simulink model "robotGrasper_FSFwInt"  (R2020a)
settings: Solver=ode45  StartTime=0.0  StopTime=tend  FixedStep=.000001  RelTol=1e-3
values from neighbouring files (symbols this model uses):
  c1 = 9982    [Robot_Grasper.m]
  c2 = -2871    [Robot_Grasper.m]
  d = 3.1    [Robot_Grasper.m]
  i_MAX = 10    [Robot_Grasper.m]
  K_FSFwInt = [Ki(1) Ki(2)]    [Robot_Grasper.m]
  Ke = -Ki(3)    [Robot_Grasper.m]
  KtKm = 1e-3*11.3    (= 0.0113)    [Robot_Grasper.m]
  m = 0.5    [Pendulum_Controller.m]    (also in Robot_Grasper.m = 0.155)
undefined symbols (not defined in the file or in its folder): a, c3
settings Model: Creator=pjseiler  LastModifiedBy=ye000064
settings DataIOCC: LimitDataPoints=on  SaveFormat=Array  ReturnWorkspaceOutputs=off
settings OptimizationCC: BlockReduction=off  BooleanDataType=off  LifeSpan=inf
settings DebuggingCC: SaveWithParameterizedLinksMsg=none  UnderspecifiedInitializationDetection=Classic  MergeDetectMultiDrivingBlocksExec=none  SignalResolutionControl=TryResolveAllWithWarning  SFUnexpectedBacktrackingDiag=warning  SFNoUnconditionalDefaultTransitionDiag=warning  SFExecutionAtInitializationDiag=none  ArithmeticOperatorsInVariantConditions=warning
settings HardwareCC: ProdBitPerPointer=32  ProdBitPerSizeT=32  ProdBitPerPtrDiffT=32  ProdLargestAtomicFloat=None  ProdIntDivRoundTo=Undefined  ProdEndianess=Unspecified  ProdWordSize=32  ProdHWDeviceType=32-bit Generic  TargetUnknown=on
settings ModelReferenceCC: PropagateSignalLabelsOutOfModel=off
settings SFSimCC: SimUseLocalCustomCode=off  CustomCodeUndefinedFunction=UseInterfaceOnly
settings RTWCC: RTWUseLocalCustomCode=off
settings CodeAppCC: StateflowObjectComments=on
settings GRTTargetCC: TargetLangStandard=C89/C90 (ANSI)
settings ConfigComp: CovMetricSettings=dw  CovHtmlReporting=on  CovSaveCumulativeToWorkspaceVar=on  CovSaveSingleToWorkspaceVar=on  CovExternalEMLEnable=off  CovSFcnEnable=off

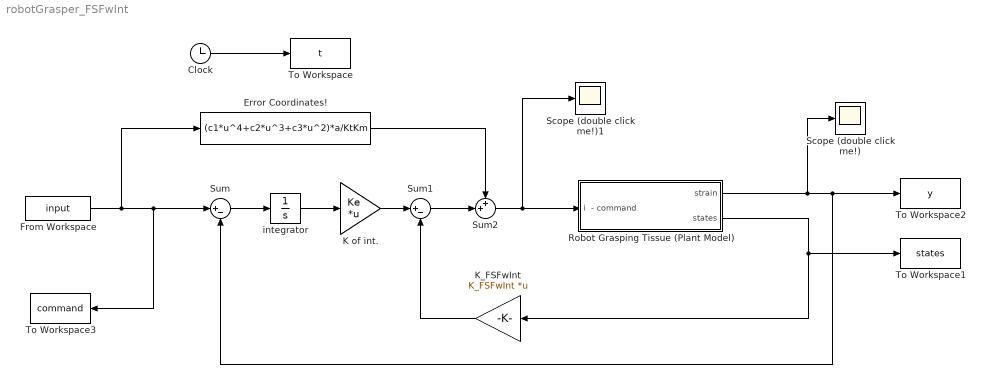
== system robotGrasper_FSFwInt ==
  Clock : Clock
  Error Coordinates! : Fcn  Expr=(c1*u^4+c2*u^3+c3*u^2)*a/KtKm
  From Workspace : FromWorkspace  VariableName=input
  K of int. : Gain  Gain=Ke  Multiplication=Matrix(K*u)
  K_FSFwInt : Gain  Gain=K_FSFwInt  Multiplication=Matrix(K*u)
  "Robot Grasping Tissue (Plant Model) " : Subsystem
  Scope (double click me!) : Scope
  Scope (double click me!)1 : Scope
  Sum : Sum  Inputs=|+-
  Sum1 : Sum  Inputs=|+-
  Sum2 : Sum  Inputs=++|
  To Workspace : ToWorkspace  VariableName=t  SampleTime=-1
  To Workspace1 : ToWorkspace  VariableName=states  SampleTime=-1
  To Workspace2 : ToWorkspace  VariableName=y  SampleTime=-1
  To Workspace3 : ToWorkspace  VariableName=command  SampleTime=-1
  integrator : Integrator
  wires:
  "Robot Grasping Tissue (Plant Model) "/1("strain ") -> To Workspace2/1, Sum/2, Scope (double click me!)/1
  Clock/1 -> To Workspace/1
  integrator/1 -> K of int./1
  Sum/1 -> integrator/1
  K of int./1 -> Sum1/1
  K_FSFwInt/1 -> Sum1/2
  "Robot Grasping Tissue (Plant Model) "/2(states) -> K_FSFwInt/1, To Workspace1/1
  From Workspace/1 -> Error Coordinates!/1, Sum/1, To Workspace3/1
  Error Coordinates!/1 -> Sum2/1
  Sum1/1 -> Sum2/2
  Sum2/1 -> Scope (double click me!)1/1, "Robot Grasping Tissue (Plant Model) "/1(i  - command)

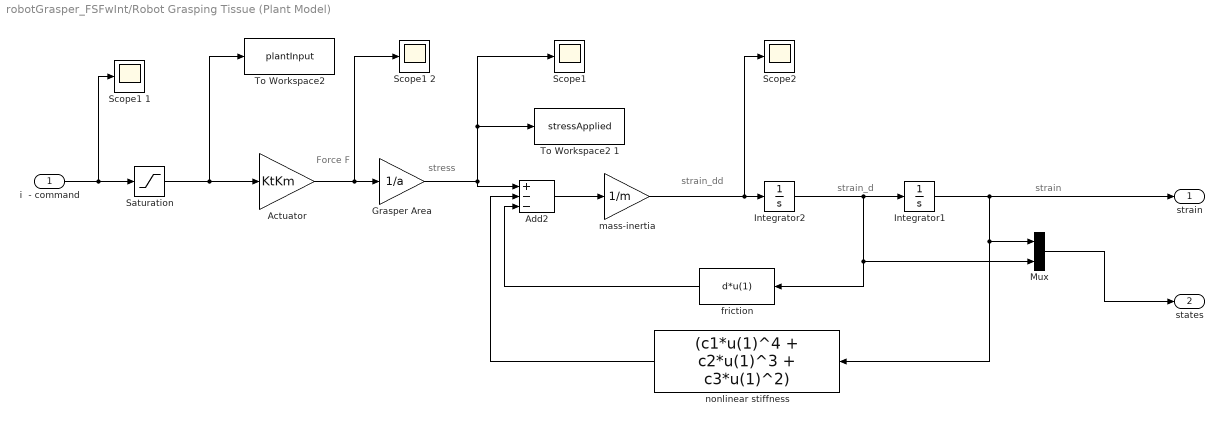
== system robotGrasper_FSFwInt/Robot Grasping Tissue (Plant Model)  ==
  note: Force F
  note: strain_d
  note: strain
  note: strain_dd
  note: stress
  i  - command : Inport
  Actuator : Gain  Gain=KtKm
  Add2 : Sum  Inputs=+--
  Grasper Area : Gain  Gain=1/a
  Integrator1 : Integrator  InitialCondition=.00001
  Integrator2 : Integrator  InitialCondition=0.000001
  Mux : Mux  Inputs=2
  Saturation : Saturate  UpperLimit=i_MAX  LowerLimit=-i_MAX
  "Scope1 " : Scope
  Scope1 1 : Scope
  Scope1 2 : Scope
  Scope2 : Scope
  "To Workspace2 " : ToWorkspace  VariableName=plantInput  SampleTime=-1
  To Workspace2 1 : ToWorkspace  VariableName=stressApplied  SampleTime=-1
  friction : Fcn  Expr=d*u(1)
  "mass-inertia " : Gain  Gain=1/m
  "nonlinear stiffness " : Fcn  Expr=(c1*u(1)^4 + c2*u(1)^3 + c3*u(1)^2)
  "strain " : Outport  VectorParamsAs1DForOutWhenUnconnected=off
  states : Outport  Port=2  VectorParamsAs1DForOutWhenUnconnected=off
  wires:
  Integrator2/1 -> Mux/2, friction/1, Integrator1/1
  Integrator1/1 -> "nonlinear stiffness "/1, Mux/1, "strain "/1
  Mux/1 -> states/1
  Add2/1 -> "mass-inertia "/1
  Actuator/1 -> Scope1 2/1, Grasper Area/1
  Saturation/1 -> "To Workspace2 "/1, Actuator/1
  i  - command/1 -> Scope1 1/1, Saturation/1
  Grasper Area/1 -> To Workspace2 1/1, "Scope1 "/1, Add2/1
  "mass-inertia "/1 -> Scope2/1, Integrator2/1
  friction/1 -> Add2/3
  "nonlinear stiffness "/1 -> Add2/2
